simulink model "untitled"  (R2012b)
settings: Solver=ode45  StartTime=0.0  StopTime=inf  RelTol=1e-3
settings Model: Creator=Vicon CS  LastModifiedBy=Vicon CS

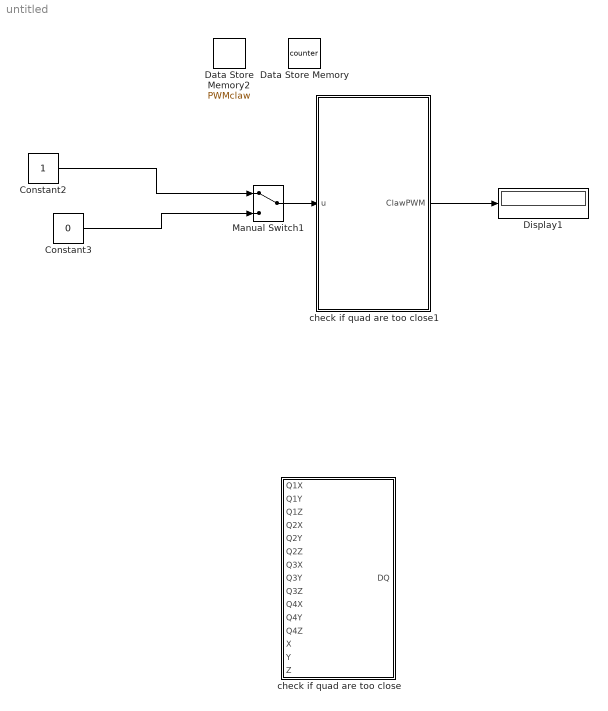
== system untitled ==
  Constant2 : Constant
  Constant3 : Constant  Value=0
  Data Store Memory : DataStoreMemory  DataStoreName=counter  InitialValue=25  OutDataTypeStr=double
  Data Store Memory2 : DataStoreMemory  DataStoreName=PWMclaw  InitialValue=1690  OutDataTypeStr=double
  Display1 : Display
  Manual Switch1 : ManualSwitch
  check if quad are too close : MATLAB Function  TreatAsAtomicUnit=on
  check if quad are too close1 : MATLAB Function  TreatAsAtomicUnit=on
  wires:
  check if quad are too close1/1(ClawPWM) -> Display1/1
  Manual Switch1/1 -> check if quad are too close1/1(u)
  Constant2/1 -> Manual Switch1/1
  Constant3/1 -> Manual Switch1/2

== matlab function untitled/check if quad are too close1 ==
  data: u input; ClawPWM output; counter data_store_memory; PWMclaw data_store_memory
function ClawPWM = CLAW(u)
global counter;
global PWMclaw;

if(u~=1)
    if(PWMclaw==1690)
        counter = 1;
        ClawPWM = PWMclaw;       
    elseif (PWMclaw==1200)
        counter = 0;
        ClawPWM = PWMclaw;
    end
    
else
    if(counter==1)
        PWMclaw = 1200;
        ClawPWM = PWMclaw;
    elseif(counter==0)
        PWMclaw = 1690;
        ClawPWM = PWMclaw;
    end
    
end

ClawPWM = PWMclaw;
   
end

== matlab function untitled/check if quad are too close ==
  data: Q1X input; Q1Y input; Q1Z input; Q2X input; Q2Y input; Q2Z input; DQ output; Q3X input; Q3Y input; Q3Z input; Q4X input; Q4Y input; Q4Z input; X input; Y input; Z input
function DQ = Distance(Q1X, Q1Y, Q1Z, Q2X, Q2Y, Q2Z, Q3X, Q3Y, Q3Z, Q4X, Q4Y, Q4Z, X, Y, Z)

DQ1 = sqrt((X-Q1X)^2 + (Y-Q1Y)^2 + (Z-Q1Z)^2);
DQ2 = sqrt((X-Q2X)^2 + (Y-Q2Y)^2 + (Z-Q2Z)^2);
DQ3 = sqrt((X-Q3X)^2 + (Y-Q3Y)^2 + (Z-Q3Z)^2);
DQ4 = sqrt((X-Q4X)^2 + (Y-Q4Y)^2 + (Z-Q4Z)^2);


if ((DQ1<1)|(DQ2<1)|(DQ3<1)|(DQ4<1))
    DQ=1;
end

end
